simulink subsystem "ROS2_Bball"  (R2024b)
settings: Solver=VariableStepAuto  StartTime=0.0  StopTime=10.0  RelTol=1e-3
settings Model: Creator=macheson  LastModifiedBy=macheson

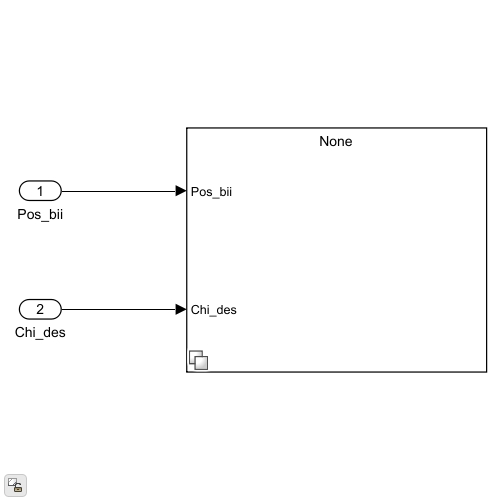
[thumbnail: Simulink's stored preview of the top-level diagram]
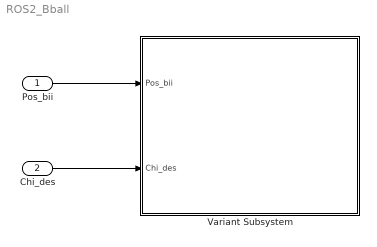
== system ROS2_Bball ==
  Pos_bii : Inport
  Chi_des : Inport  Port=2
  Variant Subsystem : Subsystem  Variant=on
  wires:
  Pos_bii/1 -> Variant Subsystem/1(Pos_bii)
  Chi_des/1 -> Variant Subsystem/2(Chi_des)

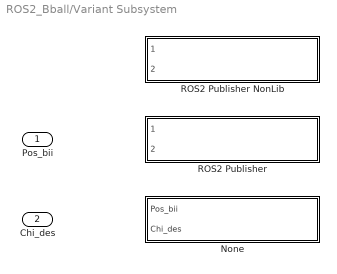
== system ROS2_Bball/Variant Subsystem ==
  Pos_bii : Inport
  Chi_des : Inport  Port=2
  None : Subsystem  VariantControl=PUB_TYPE_BBALL_NONE
  ROS2 Publisher : Subsystem  VariantControl=PUB_TYPE_BBALL_ROS2  ReferencedSubsystem=ROS2_Bball_MatPub
  ROS2 Publisher NonLib : Subsystem  VariantControl=PUB_TYPE_BBALL_ROS2_NONLIB  ReferencedSubsystem=ROS2_Bball_MatPub_NonLib

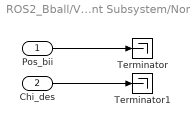
== system ROS2_Bball/Variant Subsystem/None ==
  Pos_bii : Inport
  Chi_des : Inport  Port=2
  Terminator : Terminator
  Terminator1 : Terminator
  wires:
  Pos_bii/1 -> Terminator/1
  Chi_des/1 -> Terminator1/1
